simulink model "hvac"  (R2014a)
settings: Solver=ode45  StartTime=0.0  StopTime=10.0  RelTol=1e-3
settings Model: Creator=feisele  LastModifiedBy=feisele

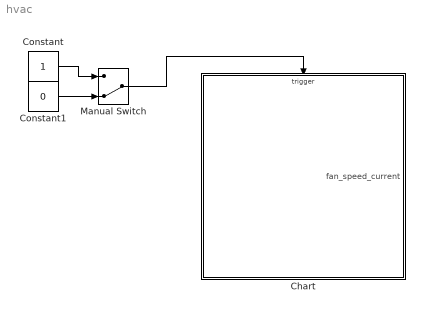
== system hvac ==
  Chart : Stateflow chart  TreatAsAtomicUnit=on
  Constant : Constant
  Constant1 : Constant  Value=0
  Manual Switch : ManualSwitch  CurrentSetting=0
  wires:
  Constant1/1 -> Manual Switch/2
  Constant/1 -> Manual Switch/1
  Manual Switch/1 -> Chart/Trigger

== stateflow chart hvac/Chart ==
  settings: executeAtInitialization=1
  state Power_off
  state Power_on
    state Fan_setting [parallel]
      settings: executionOrder=1
    state Temp_setting [parallel]
      settings: executionOrder=2
    state Mode_setting [parallel]
      settings: executionOrder=3
  Power_off -> Power_on : power_toggle {fan_speed_current = manual_fan; }
  (default) -> Power_off : { manual_fan = 5; }
  Power_on -> Power_off : [true]
  data: fan_speed_current output; manual_fan local
  events: power_toggle input RISING_EDGE_EVENT
